simulink model "analog_bp_5"  (Simulink 7.7)
settings: Solver=ode45  StartTime=0.0  StopTime=1  MaxStep=1e-4  RelTol=1e-3
values from neighbouring files (symbols this model uses):
  a = zeros(5, nord+1)    [analog_tp1.m]    (also in analog_tp2.m)
  b = fir1(nr-1,0.5)    [adapt_filter1.m]    (also in adapt_filter2.m; analog_tp1.m = zeros(5, nord+1); analog_tp2.m = zeros(5, nord+1))
undefined symbols (not defined in the file or in its folder): Fs, get
libraries: dspsnks4 x2
settings Model: Creator=svenhoffmann  LastModifiedBy=josef  ExtModeAutoUpdateStatusClock=off
settings DataIOCC: SignalLoggingName=sigsOut
settings DebuggingCC: SaveWithParameterizedLinksMsg=none  SignalResolutionControl=TryResolveAllWithWarning  SolverPrmCheckMsg=none  MultiTaskDSMMsg=warning  MultiTaskCondExecSysMsg=none  StrictBusMsg=None
settings HardwareCC: TargetUnknown=on
settings RTWCC: IncludeERTFirstTime=on

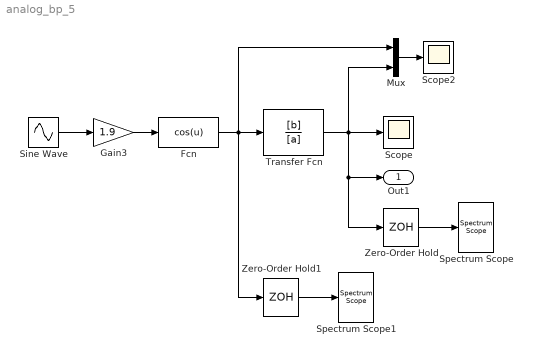
== system analog_bp_5 ==
  Fcn : Fcn  Expr=cos(u)
  Gain3 : Gain  Gain=1.9  SaturateOnIntegerOverflow=on  OutDataTypeStr=Inherit: Same as input  ParamDataTypeStr=Inherit: Same as input
  Mux : Mux  Inputs=2
  Scope : Scope
  Scope2 : Scope
      settings: YMin=0  YMax=1  SaveName=ScopeData2
  Sine Wave : Sin  Frequency=2*pi*50  SampleTime=0
  Spectrum Scope : dspsnks4/Spectrum Scope  SystemSampleTime=-1  ScopeProperties=off  Domain=Frequency  HorizSpan=1  UseBuffer=on  BufferSize=512  Overlap=64  TreatMby1Signals=M channels  inpFftLenInherit=off  FFTlength=512  numAvg=2  DisplayProperties=off  AxisGrid=on  Memory=off  FrameNumber=on  AxisLegend=off  AxisZoom=off  OpenScopeAtSimStart=on  OpenScopeImmediately=off  FigPos=get(0,'defaultfigureposition')  AxisProperties=on  XUnits=Hertz  XRange=[-Fs/2...Fs/2]  XDisplay=0  InheritXIncr=off  XIncr=1/2000  XLabel=Samples  XLimit=Auto  YUnits=dBW/Hertz  XMax=1  XMin=0  YLabel=Magnitude, dB  LineProperties=off  wintypeSpecScope=Hann  RsSpecScope=50  betaSpecScope=5  winsampSpecScope=Periodic  XAxisParamsVer=6.8  isFrameUpgraded=on
      settings: YMin=-190.8145  YMax=-8.8527
  Spectrum Scope1 : dspsnks4/Spectrum Scope  SystemSampleTime=-1  ScopeProperties=off  Domain=Frequency  HorizSpan=1  UseBuffer=on  BufferSize=512  Overlap=64  TreatMby1Signals=M channels  inpFftLenInherit=off  FFTlength=512  numAvg=2  DisplayProperties=off  AxisGrid=on  Memory=off  FrameNumber=on  AxisLegend=off  AxisZoom=off  OpenScopeAtSimStart=on  OpenScopeImmediately=off  FigPos=get(0,'defaultfigureposition')  AxisProperties=on  XUnits=Hertz  XRange=[-Fs/2...Fs/2]  XDisplay=0  InheritXIncr=off  XIncr=1/2000  XLabel=Samples  XLimit=Auto  YUnits=dBW/Hertz  XMax=1  XMin=0  YLabel=Magnitude, dB  LineProperties=off  wintypeSpecScope=Hann  RsSpecScope=50  betaSpecScope=5  winsampSpecScope=Periodic  XAxisParamsVer=6.8  isFrameUpgraded=on
      settings: YMin=-190.8145  YMax=-8.8527
  Transfer Fcn : TransferFcn  Numerator=[b]  Denominator=[a]
  Zero-Order Hold : ZeroOrderHold  SampleTime=1/2000
  Zero-Order Hold1 : ZeroOrderHold  SampleTime=1/2000
  Out1 : Outport
  wires:
  Fcn/1 -> Transfer Fcn/1, Mux/1, Zero-Order Hold1/1
  Transfer Fcn/1 -> Scope/1, Mux/2, Zero-Order Hold/1, Out1/1
  Sine Wave/1 -> Gain3/1
  Gain3/1 -> Fcn/1
  Mux/1 -> Scope2/1
  Zero-Order Hold/1 -> Spectrum Scope/1
  Zero-Order Hold1/1 -> Spectrum Scope1/1
